simulink subsystem "Bus_Generator"  (R2022a)
settings: Solver=VariableStepAuto  StartTime=0.0  StopTime=10.0  RelTol=1e-3
settings Model: Creator=ivanl  LastModifiedBy=ivanl

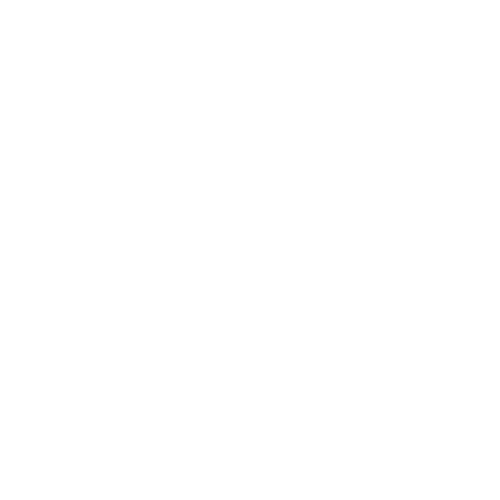
[thumbnail: Simulink's stored preview of the top-level diagram]
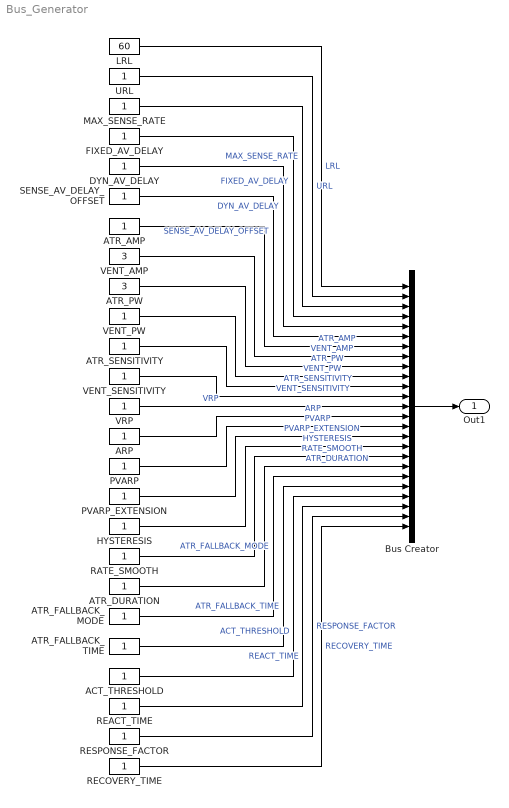
== system Bus_Generator ==
  ACT_THRESHOLD : Constant
  ARP : Constant
  ATR_AMP : Constant
  ATR_DURATION : Constant
  ATR_FALLBACK_MODE : Constant
  ATR_FALLBACK_TIME : Constant
  ATR_PW : Constant  Value=3
  ATR_SENSITIVITY : Constant
  Bus Creator : BusCreator  Inputs=25
  DYN_AV_DELAY : Constant
  FIXED_AV_DELAY : Constant
  HYSTERESIS : Constant
  LRL : Constant  Value=60
  MAX_SENSE_RATE : Constant
  PVARP : Constant
  PVARP_EXTENSION : Constant
  RATE_SMOOTH : Constant
  REACT_TIME : Constant
  RECOVERY_TIME : Constant
  RESPONSE_FACTOR : Constant
  SENSE_AV_DELAY_OFFSET : Constant
  URL : Constant
  VENT_AMP : Constant  Value=3
  VENT_PW : Constant
  VENT_SENSITIVITY : Constant
  VRP : Constant
  Out1 : Outport
  wires:
  LRL/1 -> Bus Creator/1  "LRL"
  URL/1 -> Bus Creator/2  "URL"
  MAX_SENSE_RATE/1 -> Bus Creator/3  "MAX_SENSE_RATE"
  FIXED_AV_DELAY/1 -> Bus Creator/4  "FIXED_AV_DELAY"
  DYN_AV_DELAY/1 -> Bus Creator/5  "DYN_AV_DELAY"
  SENSE_AV_DELAY_OFFSET/1 -> Bus Creator/6  "SENSE_AV_DELAY_OFFSET"
  ATR_AMP/1 -> Bus Creator/7  "ATR_AMP"
  VENT_AMP/1 -> Bus Creator/8  "VENT_AMP"
  ATR_PW/1 -> Bus Creator/9  "ATR_PW"
  VENT_PW/1 -> Bus Creator/10  "VENT_PW"
  ATR_SENSITIVITY/1 -> Bus Creator/11  "ATR_SENSITIVITY"
  VENT_SENSITIVITY/1 -> Bus Creator/12  "VENT_SENSITIVITY"
  VRP/1 -> Bus Creator/13  "VRP"
  ARP/1 -> Bus Creator/14  "ARP"
  PVARP/1 -> Bus Creator/15  "PVARP"
  PVARP_EXTENSION/1 -> Bus Creator/16  "PVARP_EXTENSION"
  HYSTERESIS/1 -> Bus Creator/17  "HYSTERESIS"
  RATE_SMOOTH/1 -> Bus Creator/18  "RATE_SMOOTH"
  ATR_DURATION/1 -> Bus Creator/19  "ATR_DURATION"
  ATR_FALLBACK_MODE/1 -> Bus Creator/20  "ATR_FALLBACK_MODE"
  ATR_FALLBACK_TIME/1 -> Bus Creator/21  "ATR_FALLBACK_TIME"
  ACT_THRESHOLD/1 -> Bus Creator/22  "ACT_THRESHOLD"
  REACT_TIME/1 -> Bus Creator/23  "REACT_TIME"
  RESPONSE_FACTOR/1 -> Bus Creator/24  "RESPONSE_FACTOR"
  RECOVERY_TIME/1 -> Bus Creator/25  "RECOVERY_TIME"
  Bus Creator/1 -> Out1/1
